simulink model "fftestSimu"  (R2014b)
settings: Solver=ode45  StartTime=0.0  StopTime=10.0  RelTol=1e-3
values from neighbouring files (symbols this model uses):
  A = [2 -3;4 -5]    [Lecture5.m]    (also in fftest.m; periodicModel.m = expm(A*Ts); test.m = [-1/(30*Ts) 0; 0 -1/(35*Ts)]; test2.m = [0      beta1   0       0)
  B = [2 3]'    [Lecture5.m]    (also in fftest.m; test.m = -A; test2.m = [0;0;0;0])
  C = [-3 2]    [Lecture5.m]    (also in fftest.m; periodicModel.m = [ones(1,numOsci*2) 1]; test.m = [1 0;0 1]; test2.m = [a1*cos(theta1) a1*sin(theta1) a2*cos(theta2) a2*sin(theta2))
  F = -place(A,B,[-3 -4])    [Lecture5.m]    (also in fftest.m; test2.m = -lqr(Ap,Bp,eye(1),eye(1)))
  L = -place(A',C',[-9 -12])'    [Lecture5.m]    (also in fftest.m; test2.m = -lqr(Ap',Cp',eye(1),eye(1))')
  M = L    [Lecture5.m]    (also in fftest.m = Mt*N; test2.m = Mt*Nc)
  N = 0    [Lecture5.m]    (also in fftest.m = -inv(Ccl/Acl*Bclt); test.m = 200; test2.m = ceil(1*24*60*60/Ts))
settings Model: Creator=rasmus  LastModifiedBy=rasmus

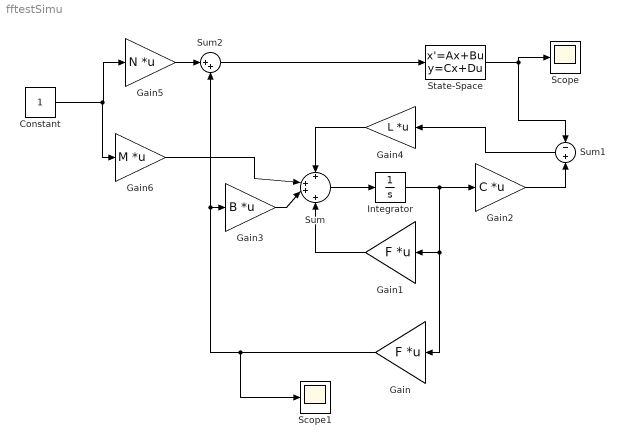
== system fftestSimu ==
  Constant : Constant
  Gain : Gain  Gain=F  Multiplication=Matrix(K*u) (u vector)
  Gain1 : Gain  Gain=F  Multiplication=Matrix(K*u) (u vector)
  Gain2 : Gain  Gain=C  Multiplication=Matrix(K*u) (u vector)
  Gain3 : Gain  Gain=B  Multiplication=Matrix(K*u) (u vector)
  Gain4 : Gain  Gain=L  Multiplication=Matrix(K*u) (u vector)
  Gain5 : Gain  Gain=N  Multiplication=Matrix(K*u) (u vector)
  Gain6 : Gain  Gain=M  Multiplication=Matrix(K*u) (u vector)
  Integrator : Integrator
  Scope : Scope
  Scope1 : Scope
  State-Space : StateSpace  A=A  B=B  C=C  D=0  X0=[0; 0]
  Sum : Sum  Inputs=+|++|+
  Sum1 : Sum  Inputs=-|+
  Sum2 : Sum  Inputs=|++
  wires:
  State-Space/1 -> Sum1/1, Scope/1
  Sum/1 -> Integrator/1
  Integrator/1 -> Gain/1, Gain1/1, Gain2/1
  Gain2/1 -> Sum1/2
  Gain/1 -> Scope1/1, Sum2/2, Gain3/1
  Sum1/1 -> Gain4/1
  Gain4/1 -> Sum/1
  Sum2/1 -> State-Space/1
  Constant/1 -> Gain6/1, Gain5/1
  Gain5/1 -> Sum2/1
  Gain1/1 -> Sum/4
  Gain3/1 -> Sum/3
  Gain6/1 -> Sum/2
